simulink model "emrax_speed_control_mode"  (R2022b)
settings: Solver=FixedStepAuto  StartTime=0.0  StopTime=2  FixedStep=1e-4  RelTol=1e-3
values from neighbouring files (symbols this model uses):
  a_fw = log(9)/trfw    [emrax_sim.m]
  ba = 2*k^2*(as*J - bm)/(np^2*psi)    [emrax_sim.m]
  bm = 0.008    [emrax_sim.m]
  I_max = I_base    [emrax_sim.m]
  J = 421e-4    (= 0.0421)    [emrax_sim.m]
  k = 1    [emrax_sim.m]
  ki_d = (ac^2)*Ld    [emrax_sim.m]
  ki_q = (ac^2)*Lq    [emrax_sim.m]
  ki_s = 2*k^2*as^2*J/(np^2*psi)    [emrax_sim.m]
  kp_d = ac*Ld    [emrax_sim.m]
  kp_q = ac*Lq    [emrax_sim.m]
  kp_s = 2*k^2*as*J/(np^2*psi)    [emrax_sim.m]
  Ld = 177*10^(-6)    (= 0.000177)    [emrax_sim.m]
  Lq = 183*10^(-6)    (= 0.000183)    [emrax_sim.m]
  max_temp = 140    [emrax_sim.m]
  np = 10    [emrax_sim.m]
  Peak_power = 50000    [emrax_sim.m]
  Peak_regen = -1500000    [emrax_sim.m]
  psi = 0.0542*k    (= 0.0542)    [emrax_sim.m]
  Ra_d = ac*Ld-Rs    [emrax_sim.m]
  Ra_q = ac*Lq-Rs    [emrax_sim.m]
  rpm_nom = 5100    [emrax_sim.m]
  Rs = 18e-3    (= 0.018)    [emrax_sim.m]
  temp_threshold = 100    [emrax_sim.m]
  u_dc = 550    [emrax_sim.m]
  u_nom = u_dc*k    (= 550)    [emrax_sim.m]
  Vd_lim = u_nom    (= 550)    [emrax_sim.m]
libraries: simulink x6, spsMeanLib x1, spspowerguiLib x1
settings Model: Creator=alexa  LastModifiedBy=alexa

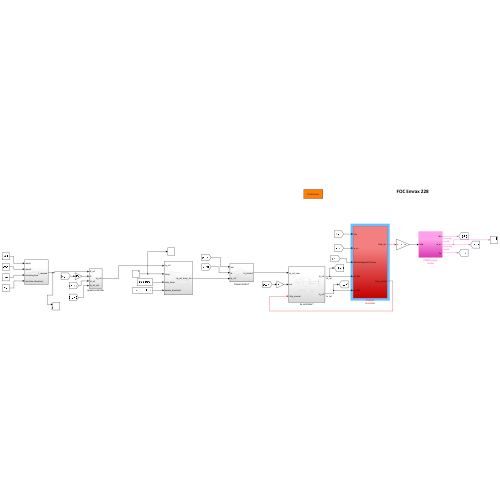
[thumbnail: Simulink's stored preview of the top-level diagram]
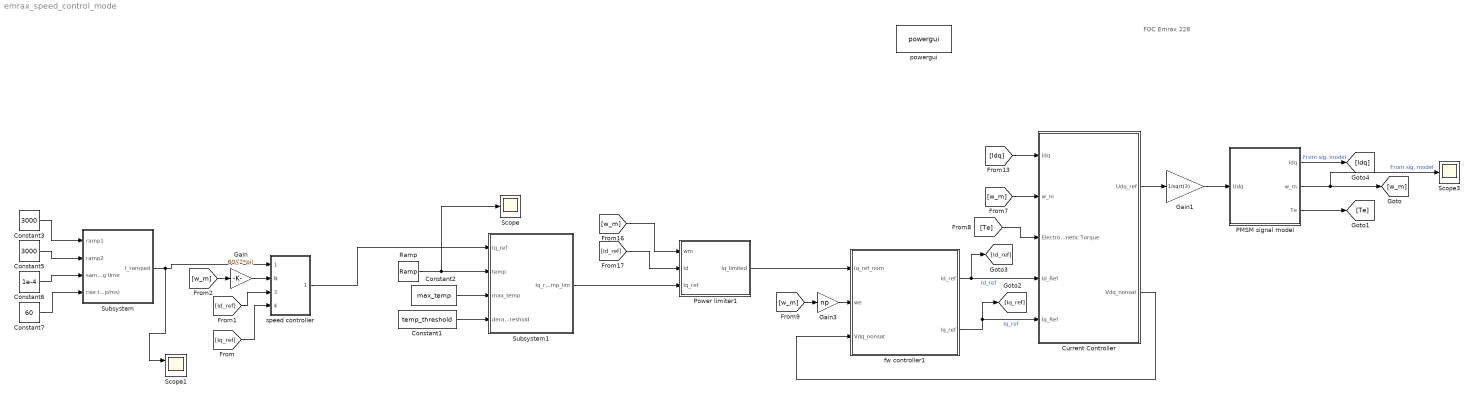
== system emrax_speed_control_mode ==
  note: FOC Emrax 228
  Constant1 : Constant  Value=temp_threshold
  Constant2 : Constant  Value=max_temp
  Constant3 : Constant  Value=3000
  Constant5 : Constant  Value=3000
  Constant6 : Constant  Value=1e-4
  Constant7 : Constant  Value=60
  Current Controller : Subsystem
  Gain : Gain  Gain=60/(2*pi)
  Gain1 : Gain  Gain=1/sqrt(3)
  Gain3 : Gain  Gain=np
  PMSM signal model : Subsystem
  Power limiter1 : Subsystem
  Ramp : simulink/Sources/Ramp  slope=1  start=0  InitialOutput=30
  Scope : Scope
  Scope1 : Scope  NumInputPorts=2
  Scope3 : Scope
  Subsystem : Subsystem
  Subsystem1 : Subsystem
  fw controller1 : Subsystem
  powergui : spspowerguiLib/powergui  Priority=1  SimulationMode=Continuous  SampleTime=50e-6  frequency=60  Iterations=50  frequencyindice=0  Pbase=100e6  ErrMax=1e-4  UnitsV=kV  UnitsW=MW  buscounter=0  FunctionMessages=off  echomessages=off  EnableUseOfTLC=off  CurrentSourceSwitches=off  DisableSnubberDevices=off  DisableRonSwitches=off  DisableVfSwitches=off  DisplayEquations=off  AutomaticDiscreteSolvers=off  SolverType=Tustin/Backward Euler (TBE)  Interpol=off  ExternalGateDelay=off  methode=off  Ts=100  x0status=blocks  SPID=on  SwTol=0  HookPort=off  NonlinearTolerance=0  nMaxIteration=15  ContinueOnMaxIteration=off  RestoreLinks=warning  ResistiveCurrentMeasurement=off  Frange=[0:2:500]  Ylog=off  Xlog=on  ShowGrid=off  save=off  variable=ZData  structure=0  ZoomFFT=off  StartTime=0.0  cycles=1  DisplayStyle=1  fundamental=60  FreqAxis=off  MaxFrequency=1000  frequencyindicesteady=1  RmsSteady=1  display=off
  speed controller : Subsystem
  wires:
  fw controller1/2(Iq_ref) -> Current Controller/5(Iq_Ref), [Iq_ref]  "Iq_ref"
  Gain3/1 -> fw controller1/2(we)
  Constant7/1 -> Subsystem/4(rise time (Amp/ms))
  Constant6/1 -> Subsystem/3(sampling time)
  PMSM signal model/3("Te ") -> [Te]
  [Te] -> Current Controller/3(Electromagnetic Torque)
  [w_m] -> Gain3/1
  [w_m] -> Current Controller/2(w_m)
  PMSM signal model/1(Idq) -> [Idq]  "From sig. model"
  Gain1/1 -> PMSM signal model/1(Udq)
  Constant5/1 -> Subsystem/2(ramp2)
  Current Controller/2(Vdq_nonsat) -> fw controller1/3(Vdq_nonsat)
  [Idq] -> Current Controller/1(Idq)
  fw controller1/1(Id_ref) -> Current Controller/4(Id_Ref), [Id_ref]  "Id_ref"
  Current Controller/1("Udq_ref ") -> Gain1/1
  PMSM signal model/2("w_m ") -> [w_m], Scope3/1  "From sig. model"
  Constant3/1 -> Subsystem/1(ramp1)
  [w_m] -> Power limiter1/1(wm)
  [Id_ref] -> Power limiter1/2(Id)
  [Iq_ref] -> speed controller/4(Iq_ref_sat)
  [Id_ref] -> speed controller/3(Id_ref)
  Gain/1 -> speed controller/2(N)
  [w_m] -> Gain/1
  Power limiter1/1(Iq_limited) -> fw controller1/1(Iq_ref_nom)
  Constant1/1 -> Subsystem1/4(derate_threshold)
  Constant2/1 -> Subsystem1/3(max_temp)
  Ramp/1 -> Scope/1, Subsystem1/2(temp)
  Subsystem1/1(Iq_ref_temp_lim) -> Power limiter1/3(Iq_ref)
  speed controller/1(Iq_ref) -> Subsystem1/1(Iq_ref)
  Subsystem/1(I_ramped) -> Scope1/1, speed controller/1(N_ref)

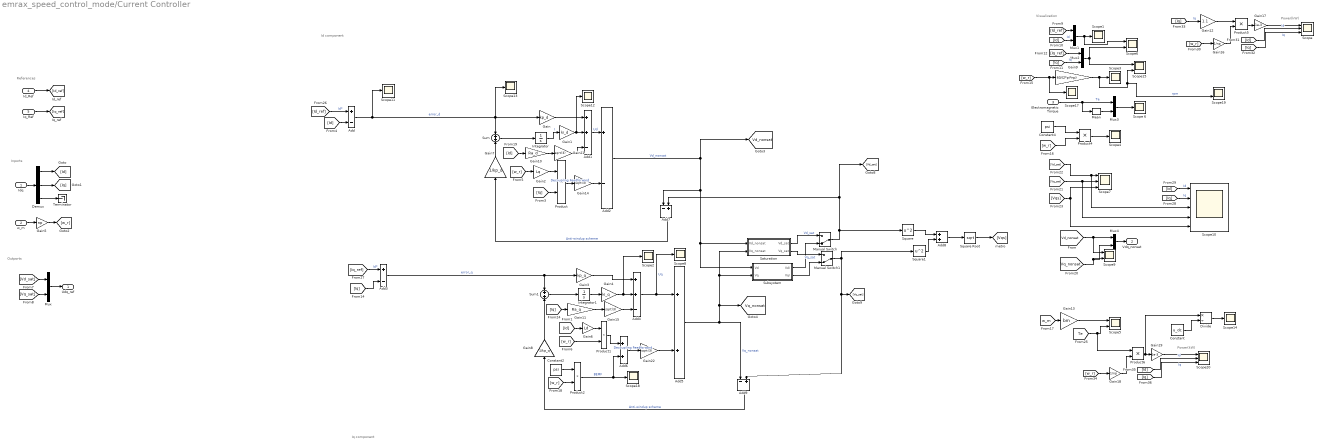
== system emrax_speed_control_mode/Current Controller ==
  note: Power(kW)
  note: References
  note: Id component
  note: Iq component
  note: Inports
  note: Outports
  note: Visualization
  note: Power(kW)
  Idq : Inport
  w_m : Inport  Port=2
  Electromagnetic Torque : Inport  Port=3
  Id_Ref : Inport  Port=4
  Iq_Ref : Inport  Port=5
  Add : Sum  Inputs=+-
  Add1 : Sum  Inputs=++-
  Add2 : Sum  Inputs=+-
  Add3 : Sum  Inputs=+-
  Add4 : Sum  Inputs=++-
  Add5 : Sum
  Add6 : Sum
  Add7 : Sum  Inputs=-+
  Add8 : Sum
  Add9 : Sum  Inputs=-+
  Constant : Constant  Value=u_dc
  Constant2 : Constant  Value=psi
  Constant4 : Constant  Value=psi
  Demux : Demux  Outputs=3
  Divide : Product  Inputs=*/
  Gain : Gain  Gain=kp_d
  Gain1 : Gain  Gain=ki_d
  Gain10 : Gain  Gain=Ra_d
  Gain11 : Gain  Gain=Ra_q
  Gain12 : Gain  Gain=1.1
  Gain13 : Gain  Gain=bm
  Gain{14..15,21..22} (4 alike) : Gain  Gain=sqrt(3)
  Gain16 : Gain  Gain=1/np
  Gain17 : Gain  Gain=1e-3
  Gain18 : Gain  Gain=1/np
  Gain19 : Gain  Gain=1e-3
  Gain2 : Gain  Gain=Lq
  Gain3 : Gain  Gain=kp_q
  Gain4 : Gain  Gain=ki_q
  Gain5 : Gain  Gain=np
  Gain6 : Gain  Gain=Ld
  Gain7 : Gain  Gain=1/kp_d
  Gain8 : Gain  Gain=1/kp_q
  Gain9 : Gain  Gain=60/(2*pi*np)
  Integrator : Integrator
  Integrator1 : Integrator
  Manual Switch : ManualSwitch  CurrentSetting=0
  Manual Switch1 : ManualSwitch  CurrentSetting=0
  Mean : spsMeanLib/Mean  Freq=fsw  Vinit=0  Ts=0
  Mux{,1..4} (5 alike) : Mux  Inputs=2
  Product{,1..2,4..6} (6 alike) : Product
  Saturation : Subsystem
  Scope : Scope  NumInputPorts=3
  Scope 6 : Scope
  Scope{1..4,8,11..14,17..18} (11 alike) : Scope
  Scope10 : Scope  NumInputPorts=5
  Scope{5..6,9,15,19} (5 alike) : Scope  NumInputPorts=2
  Scope20 : Scope  NumInputPorts=3
  Scope7 : Scope  NumInputPorts=3
  Square : Math  Operator=square
  Square Root : Sqrt
  Square1 : Math  Operator=square
  Subsystem : Subsystem
  Sum : Sum
  Sum1 : Sum
  Terminator : Terminator
  "Udq_ref " : Outport  VectorParamsAs1DForOutWhenUnconnected=off
  Vdq_nonsat : Outport  Port=2
  tag scope: Vd_nonsat=global, Vq_nonsat=global
  wires:
  Gain4/1 -> Scope2/1, Add4/2
  [Id] -> Gain6/1
  Add4/1 -> Scope8/1, Add5/1  "Uq"
  Add1/1 -> Add2/1  "Ud"
  [w_r] -> Gain2/1
  Gain2/1 -> Product/1
  Gain3/1 -> Add4/1
  [Iq] -> Product/2
  Integrator/1 -> Gain1/1  "I"
  Sum/1 -> Integrator/1
  Gain/1 -> Add1/1
  [w_r] -> Product1/2
  Gain6/1 -> Product1/1
  Idq/1 -> Demux/1
  Product/1 -> Gain14/1  "Decoupling Feedforward"
  Gain7/1 -> Sum/2
  Add2/1 -> [Vd_nonsat], Saturation/1(Vd_nonsat), Subsystem/1(Vd), Add7/1  "Vd_nonsat"
  Add7/1 -> Gain7/1  "Anti-windup scheme"
  Sum1/1 -> Integrator1/1
  Add5/1 -> Add9/1, Subsystem/2(Vq), Saturation/2(Vq_nonsat), [Vq_nonsat]  "Vq_nonsat"
  Gain8/1 -> Sum1/2
  Add9/1 -> Gain8/1  "Anti-windup scheme"
  Demux/1 -> [Id]
  Demux/2 -> [Iq]
  Demux/3 -> Terminator/1
  w_m/1 -> Gain5/1
  Gain5/1 -> [w_r]
  [Vd_sat] -> Mux/1
  [Vq_sat] -> Mux/2
  Mux/1 -> "Udq_ref "/1
  [Id] -> Add/2
  Mux1/1 -> Scope6/1, Scope1/1
  [Id_ref] -> Mux1/1
  [Id] -> Mux1/2  "Id"
  [Iq_ref] -> Mux2/1
  [Iq] -> Mux2/2  "Iq"
  [w_r] -> Scope17/1, Gain9/1
  Gain9/1 -> Scope19/2, Scope15/2, Scope3/1  "rpm"
  Mux3/1 -> Scope 6/1
  Electromagnetic Torque/1 -> Mean/1, Mux3/1  "Te"
  Mean/1 -> Mux3/2
  Constant2/1 -> Product2/1
  Product1/1 -> Add6/1
  Add6/1 -> Gain22/1  "Decoupling Feedforward"
  Add/1 -> Scope11/1, Gain/1, Sum/1, Scope13/1  "error_d"
  Add3/1 -> Sum1/1, Gain3/1  "error_q"
  [Iq] -> Add3/2
  Gain1/1 -> Scope12/1, Add1/2
  Integrator1/1 -> Gain4/1
  Square1/1 -> Add8/2
  Square/1 -> Add8/1
  Add8/1 -> Square Root/1
  [Vd_nonsat] -> Scope9/1, Mux4/1
  [Vq_nonsat] -> Mux4/2, Scope9/2
  Square Root/1 -> [Vqs]
  [Vd_sat] -> Scope10/3, Scope7/1
  [Vq_sat] -> Scope10/4, Scope7/2
  [Vqs] -> Scope7/3, Scope10/5
  [Id] -> Gain10/1
  [Iq] -> Gain11/1
  [w_r] -> Product4/2
  Constant4/1 -> Product4/1
  Product4/1 -> Scope4/1
  Id_Ref/1 -> [Id_ref]
  Iq_Ref/1 -> [Iq_ref]
  Gain13/1 -> Scope5/1
  [Te] -> Product6/1, Scope5/2
  [w_m] -> Gain13/1
  Gain12/1 -> Product5/1
  Mux2/1 -> Scope6/2, Scope15/1
  [Iq] -> Scope10/2  "Iq"
  [Id] -> Scope10/1  "Id"
  [Id_ref] -> Add/1  "Id*"
  Subsystem/1(Vd\) -> Manual Switch/2
  Saturation/1(Vd_sat) -> Manual Switch/1  "Vd_sat"
  Saturation/2(Vq_sat) -> Manual Switch1/1  "Vq_sat"
  Subsystem/2(Vq\) -> Manual Switch1/2
  Manual Switch/1 -> Square/1, [Vd_sat], Add7/2
  Manual Switch1/1 -> [Vq_sat], Add9/2, Square1/1
  Gain11/1 -> Gain15/1
  [w_r] -> Product2/2
  Product2/1 -> Scope18/1, Add6/2  "BEMF"
  Mux4/1 -> Vdq_nonsat/1
  [Iq_ref] -> Add3/1  "Id*"
  Product5/1 -> Gain17/1
  [w_r] -> Gain16/1
  Gain16/1 -> Product5/2
  [Id] -> Scope/2  "Id"
  [Iq] -> Scope/3  "Iq"
  [Iq] -> Gain12/1  "Iq"
  Gain17/1 -> Scope/1
  Gain19/1 -> Scope20/1
  [Iq] -> Scope20/3  "Iq"
  [Id] -> Scope20/2  "Id"
  Gain18/1 -> Product6/2
  Product6/1 -> Divide/1, Gain19/1
  [w_r] -> Gain18/1
  Gain15/1 -> Add4/3
  Gain10/1 -> Gain21/1
  Gain21/1 -> Add1/3
  Gain14/1 -> Add2/2
  Gain22/1 -> Add5/2
  Constant/1 -> Divide/2
  Divide/1 -> Scope14/1

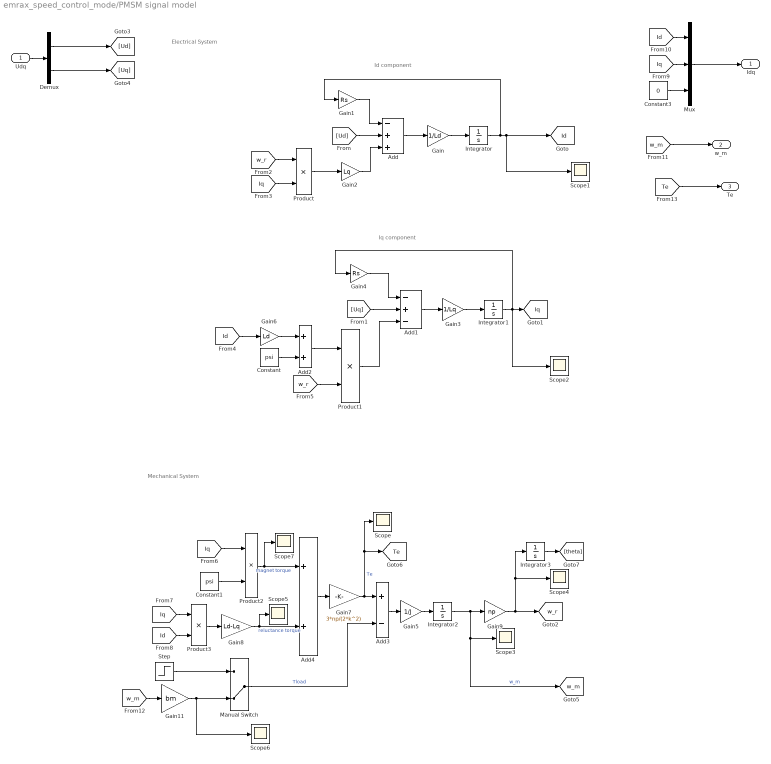
== system emrax_speed_control_mode/PMSM signal model ==
  note: Electrical System
  note: Id component
  note: Iq component
  note: Mechanical System
  Udq : Inport
  Add : Sum  Inputs=-++
  Add1 : Sum  Inputs=-+-
  Add2 : Sum
  Add3 : Sum  Inputs=+-
  Add4 : Sum
  Constant : Constant  Value=psi
  Constant1 : Constant  Value=psi
  Constant3 : Constant  Value=0
  Demux : Demux  Outputs=2
  Gain : Gain  Gain=1/Ld
  Gain1 : Gain  Gain=Rs
  Gain11 : Gain  Gain=bm
  Gain2 : Gain  Gain=Lq
  Gain3 : Gain  Gain=1/Lq
  Gain4 : Gain  Gain=Rs
  Gain5 : Gain  Gain=1/J
  Gain6 : Gain  Gain=Ld
  Gain7 : Gain  Gain=3*np/(2*k^2)
  Gain8 : Gain  Gain=Ld-Lq
  Gain9 : Gain  Gain=np
  Integrator{,1..3} (4 alike) : Integrator
  Manual Switch : ManualSwitch  CurrentSetting=0
  Mux : Mux  Inputs=3
  Product{,1..3} (4 alike) : Product
  Scope{,1..7} (8 alike) : Scope
  Step : Step  Time=0.5  After=200  SampleTime=0
  Idq : Outport  VectorParamsAs1DForOutWhenUnconnected=off
  "w_m " : Outport  Port=2  VectorParamsAs1DForOutWhenUnconnected=off
  "Te " : Outport  Port=3  VectorParamsAs1DForOutWhenUnconnected=off
  tag scope: Id=global, Iq=global, Te=global, w_m=global, w_r=global
  wires:
  Add3/1 -> Gain5/1
  Add2/1 -> Product1/1
  Product/1 -> Gain2/1
  Gain/1 -> Integrator/1
  Integrator1/1 -> Scope2/1, [Iq], Gain4/1
  Gain6/1 -> Add2/1
  Gain1/1 -> Add/1
  Product3/1 -> Gain8/1
  Integrator/1 -> Gain1/1, Scope1/1, [Id]
  Gain8/1 -> Add4/2, Scope5/1  "reluctance torque"
  Gain5/1 -> Integrator2/1
  Gain7/1 -> Add3/1, [Te], Scope/1  "Te"
  Constant1/1 -> Product2/2
  Add4/1 -> Gain7/1
  [Iq] -> Product3/1
  Product2/1 -> Add4/1, Scope7/1  "magnet torque"
  [Iq] -> Product2/1
  Gain2/1 -> Add/3
  [w_r] -> Product/1
  [Id] -> Gain6/1
  [Iq] -> Product/2
  Gain3/1 -> Integrator1/1
  [w_r] -> Product1/2
  Constant/1 -> Add2/2
  Gain4/1 -> Add1/1
  Product1/1 -> Add1/3
  Add1/1 -> Gain3/1
  [Ud] -> Add/2
  Add/1 -> Gain/1
  [Uq] -> Add1/2
  [Id] -> Product3/2
  Udq/1 -> Demux/1
  Integrator2/1 -> Gain9/1, [w_m], Scope3/1  "w_m"
  Gain9/1 -> Scope4/1, Integrator3/1, [w_r]
  Manual Switch/1 -> Add3/2  "Tload"
  Step/1 -> Manual Switch/1
  [w_m] -> Gain11/1
  [Id] -> Mux/1
  [Iq] -> Mux/2
  [w_m] -> "w_m "/1
  Constant3/1 -> Mux/3
  [Te] -> "Te "/1
  Integrator3/1 -> [theta]
  Demux/1 -> [Ud]
  Demux/2 -> [Uq]
  Mux/1 -> Idq/1
  Gain11/1 -> Scope6/1, Manual Switch/2

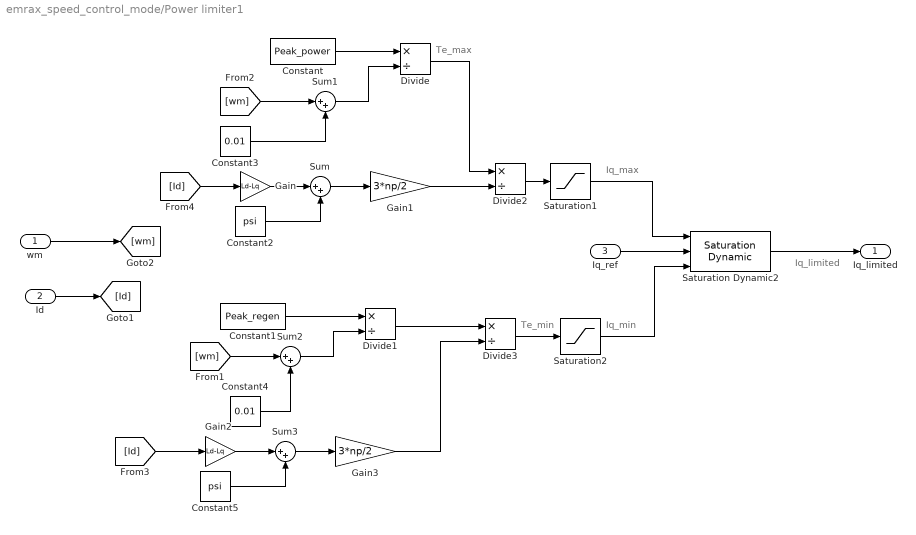
== system emrax_speed_control_mode/Power limiter1 ==
  note: Te_max
  note: Iq_limited
  note: Iq_max
  note: Iq_min
  note: Te_min
  wm : Inport
  Id : Inport  Port=2
  Iq_ref : Inport  Port=3
  Constant : Constant  Value=Peak_power
  Constant1 : Constant  Value=Peak_regen
  Constant2 : Constant  Value=psi
  Constant3 : Constant  Value=0.01
  Constant4 : Constant  Value=0.01
  Constant5 : Constant  Value=psi
  Divide{,1..3} (4 alike) : Product  Inputs=*/
  Gain : Gain  Gain=Ld-Lq
  Gain1 : Gain  Gain=3*np/2
  Gain2 : Gain  Gain=Ld-Lq
  Gain3 : Gain  Gain=3*np/2
  Saturation Dynamic2 : simulink/Discontinuities/Saturation Dynamic  OutMin=[]  OutMax=[]  OutDataTypeStr=Inherit: Same as second input  OutDataType=fixdt(1, 16)  OutScaling=2^-10  DoSatur=off
  Saturation1 : Saturate  UpperLimit=10000  LowerLimit=-10000
  Saturation2 : Saturate  UpperLimit=10000  LowerLimit=-10000
  Sum{,1..3} (4 alike) : Sum  Inputs=|++
  Iq_limited : Outport
  wires:
  Sum2/1 -> Divide1/2
  [wm] -> Sum2/1
  Constant4/1 -> Sum2/2
  Saturation2/1 -> Saturation Dynamic2/3
  Saturation1/1 -> Saturation Dynamic2/1
  Constant3/1 -> Sum1/2
  [wm] -> Sum1/1
  Sum1/1 -> Divide/2
  Divide2/1 -> Saturation1/1
  Divide3/1 -> Saturation2/1
  Divide/1 -> Divide2/1
  Constant1/1 -> Divide1/1
  Constant/1 -> Divide/1
  Divide1/1 -> Divide3/1
  Saturation Dynamic2/1 -> Iq_limited/1
  wm/1 -> [wm]
  Iq_ref/1 -> Saturation Dynamic2/2
  Gain1/1 -> Divide2/2
  Gain/1 -> Sum/1
  Constant2/1 -> Sum/2
  Sum/1 -> Gain1/1
  Sum3/1 -> Gain3/1
  [Id] -> Gain2/1
  Gain2/1 -> Sum3/1
  Constant5/1 -> Sum3/2
  Gain3/1 -> Divide3/2
  Id/1 -> [Id]
  [Id] -> Gain/1

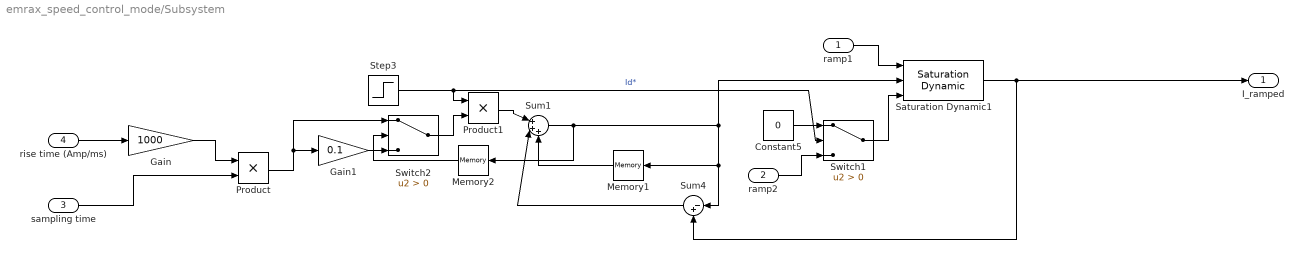
== system emrax_speed_control_mode/Subsystem ==
  ramp1 : Inport
  ramp2 : Inport  Port=2
  sampling time : Inport  Port=3
  rise time (Amp/ms) : Inport  Port=4
  Constant5 : Constant  Value=0
  Gain : Gain  Gain=1000
  Gain1 : Gain  Gain=0.1
  Memory1 : Memory
  Memory2 : Memory
  Product : Product
  Product1 : Product
  Saturation Dynamic1 : simulink/Discontinuities/Saturation Dynamic  OutMin=[]  OutMax=[]  OutDataTypeStr=Inherit: Same as second input  OutDataType=fixdt(1, 16)  OutScaling=2^-10  DoSatur=off
  Step3 : Step  Time=2  Before=1  After=-1  SampleTime=0
  Sum1 : Sum  Inputs=|+++
  Sum4 : Sum  Inputs=|-+
  Switch1 : Switch  Criteria=u2 > Threshold  SaturateOnIntegerOverflow=off  InputSameDT=off
  Switch2 : Switch  Criteria=u2 > Threshold  SaturateOnIntegerOverflow=off  InputSameDT=off
  I_ramped : Outport
  wires:
  Sum1/1 -> Memory2/1, Sum4/1, Memory1/1, Saturation Dynamic1/2
  Switch2/1 -> Product1/2
  Memory2/1 -> Switch2/2
  Product1/1 -> Sum1/1
  Memory1/1 -> Sum1/3
  Gain1/1 -> Switch2/3
  Switch1/1 -> Saturation Dynamic1/3
  Step3/1 -> Switch1/2, Product1/1  "Id*"
  Sum4/1 -> Sum1/2
  Constant5/1 -> Switch1/1
  Saturation Dynamic1/1 -> Sum4/2, I_ramped/1
  ramp2/1 -> Switch1/3
  ramp1/1 -> Saturation Dynamic1/1
  rise time (Amp/ms)/1 -> Gain/1
  sampling time/1 -> Product/2
  Gain/1 -> Product/1
  Product/1 -> Switch2/1, Gain1/1

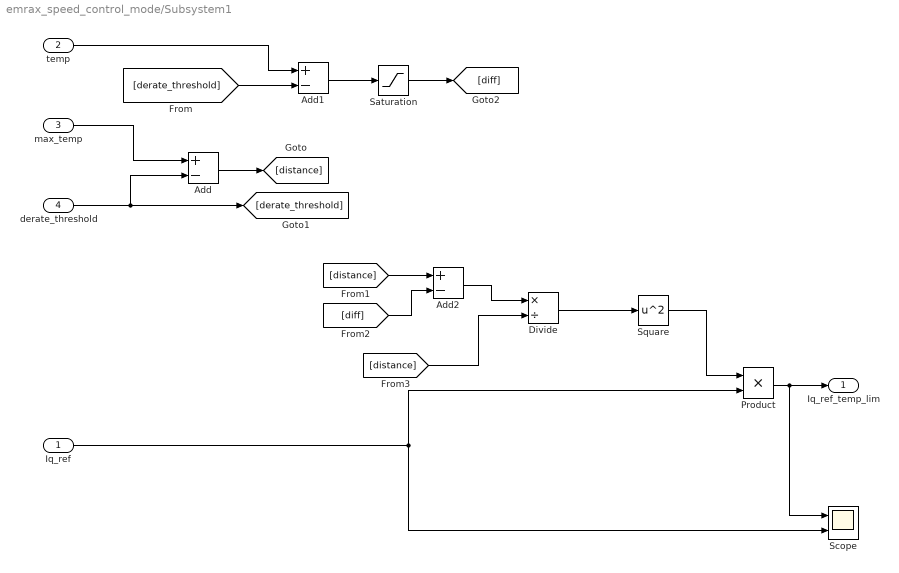
== system emrax_speed_control_mode/Subsystem1 ==
  Iq_ref : Inport
  temp : Inport  Port=2
  max_temp : Inport  Port=3
  derate_threshold : Inport  Port=4
  Add : Sum  Inputs=+-
  Add1 : Sum  Inputs=+-
  Add2 : Sum  Inputs=+-
  Divide : Product  Inputs=*/
  Product : Product
  Saturation : Saturate  UpperLimit=1000  LowerLimit=0
  Scope : Scope  NumInputPorts=2
  Square : Math  Operator=square
  Iq_ref_temp_lim : Outport
  wires:
  max_temp/1 -> Add/1
  Add/1 -> [distance]
  derate_threshold/1 -> [derate_threshold], Add/2
  [derate_threshold] -> Add1/2
  temp/1 -> Add1/1
  Add1/1 -> Saturation/1
  Saturation/1 -> [diff]
  [distance] -> Add2/1
  [diff] -> Add2/2
  Add2/1 -> Divide/1
  [distance] -> Divide/2
  Divide/1 -> Square/1
  Iq_ref/1 -> Product/2, Scope/2
  Square/1 -> Product/1
  Product/1 -> Scope/1, Iq_ref_temp_lim/1

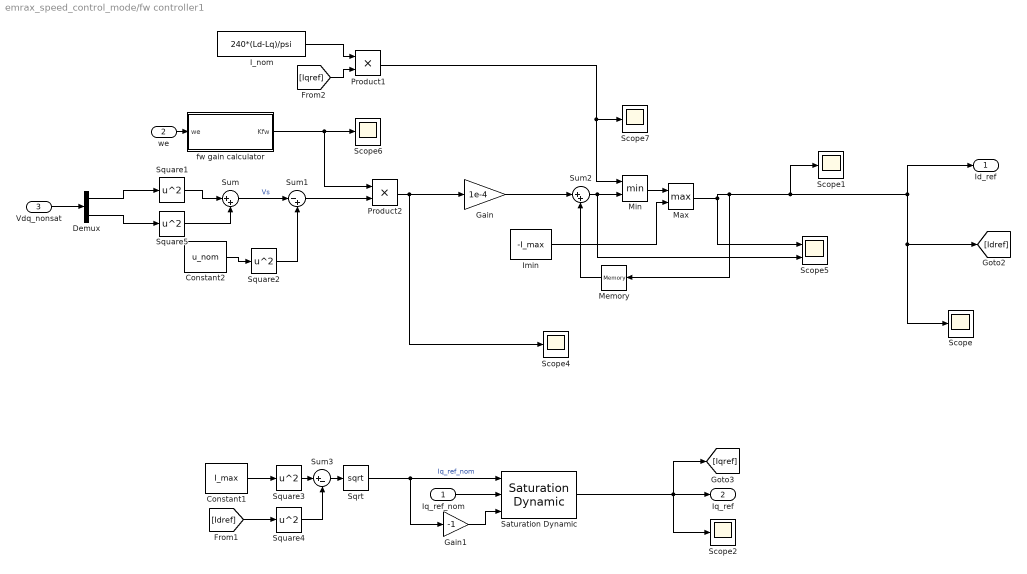
== system emrax_speed_control_mode/fw controller1 ==
  Iq_ref_nom : Inport
  we : Inport  Port=2
  Vdq_nonsat : Inport  Port=3
  Constant1 : Constant  Value=I_max
  Constant2 : Constant  Value=u_nom
  Demux : Demux  Outputs=2
  Gain : Gain  Gain=1e-4
  Gain1 : Gain  Gain=-1
  I_nom : Constant  Value=240*(Ld-Lq)/psi
  Imin : Constant  Value=-I_max
  Max : MinMax  Function=max  Inputs=2
  Memory : Memory
  Min : MinMax  Inputs=2
  Product1 : Product
  Product2 : Product
  Saturation Dynamic : simulink/Discontinuities/Saturation Dynamic  OutMin=[]  OutMax=[]  OutDataTypeStr=Inherit: Same as second input  OutDataType=fixdt(1, 16)  OutScaling=2^-10  DoSatur=off
  Scope{,1..2,4,6..7} (6 alike) : Scope
  Scope5 : Scope  NumInputPorts=2
  Sqrt : Sqrt
  Square{1..5} (5 alike) : Math  Operator=square
  Sum : Sum  Inputs=|++
  Sum1 : Sum  Inputs=|-+
  Sum2 : Sum  Inputs=|++
  Sum3 : Sum  Inputs=|+-
  fw gain calculator : Subsystem
  Id_ref : Outport
  Iq_ref : Outport  Port=2
  wires:
  Max/1 -> Scope5/1, Memory/1, Scope1/1, [Idref], Scope/1, Id_ref/1
  Product2/1 -> Scope4/1, Gain/1
  Sum1/1 -> Product2/2
  fw gain calculator/1(Kfw) -> Scope6/1, Product2/1
  [Iqref] -> Product1/2
  [Idref] -> Square4/1
  Square5/1 -> Sum/2
  Square1/1 -> Sum/1
  Vdq_nonsat/1 -> Demux/1
  Demux/1 -> Square1/1
  Demux/2 -> Square5/1
  I_nom/1 -> Product1/1
  Gain1/1 -> Saturation Dynamic/3
  Imin/1 -> Max/2
  Sum3/1 -> Sqrt/1
  Constant2/1 -> Square2/1
  Sum/1 -> Sum1/1  "Vs"
  Square2/1 -> Sum1/2
  we/1 -> fw gain calculator/1(we)
  Constant1/1 -> Square3/1
  Square3/1 -> Sum3/1
  Square4/1 -> Sum3/2
  Iq_ref_nom/1 -> Saturation Dynamic/2
  Sqrt/1 -> Saturation Dynamic/1, Gain1/1  "Iq_ref_nom"
  Saturation Dynamic/1 -> Scope2/1, Iq_ref/1, [Iqref]
  Gain/1 -> Sum2/1
  Sum2/1 -> Min/2, Scope5/2
  Memory/1 -> Sum2/2
  Product1/1 -> Min/1, Scope7/1
  Min/1 -> Max/1

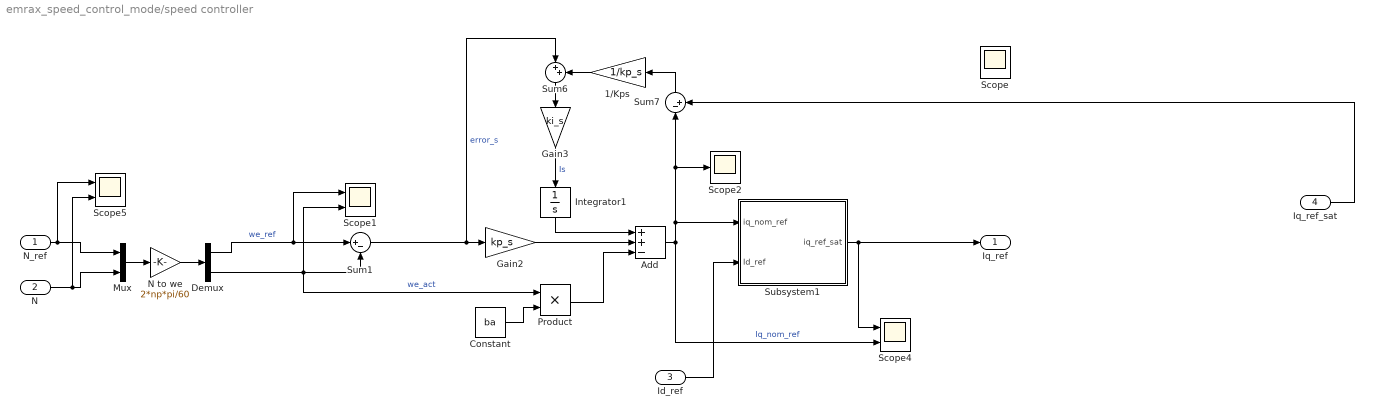
== system emrax_speed_control_mode/speed controller ==
  N_ref : Inport
  N : Inport  Port=2
  Id_ref : Inport  Port=3
  Iq_ref_sat : Inport  Port=4
  1/Kps : Gain  Gain=1/kp_s
  Add : Sum  Inputs=++-
  Constant : Constant  Value=ba
  Demux : Demux  Outputs=2
  Gain2 : Gain  Gain=kp_s
  Gain3 : Gain  Gain=ki_s
  Integrator1 : Integrator
  Mux : Mux  Inputs=2
  N to we : Gain  Gain=2*np*pi/60
  Product : Product
  Scope : Scope
  Scope1 : Scope  NumInputPorts=2
  Scope2 : Scope
  Scope4 : Scope  NumInputPorts=2
  Scope5 : Scope  NumInputPorts=2
  Subsystem1 : Subsystem
  Sum1 : Sum  Inputs=|+-
  Sum6 : Sum  Inputs=|++
  Sum7 : Sum  Inputs=|-+
  Iq_ref : Outport
  wires:
  Sum7/1 -> 1/Kps/1
  Add/1 -> Scope2/1, Sum7/1, Subsystem1/1(iq_nom_ref), Scope4/2  "Iq_nom_ref"
  Gain2/1 -> Add/2
  1/Kps/1 -> Sum6/2
  Sum1/1 -> Gain2/1, Sum6/1  "error_s"
  N_ref/1 -> Scope5/1, Mux/1
  N/1 -> Scope5/2, Mux/2
  Constant/1 -> Product/2
  Gain3/1 -> Integrator1/1  "Is"
  Product/1 -> Add/3
  Demux/1 -> Scope1/1, Sum1/1  "we_ref"
  Demux/2 -> Product/1, Sum1/2, Scope1/2  "we_act"
  Sum6/1 -> Gain3/1
  Subsystem1/1(iq_ref_sat) -> Scope4/1, Iq_ref/1
  Mux/1 -> N to we/1
  N to we/1 -> Demux/1
  Integrator1/1 -> Add/1
  Id_ref/1 -> Subsystem1/2(Id_ref)
  Iq_ref_sat/1 -> Sum7/2

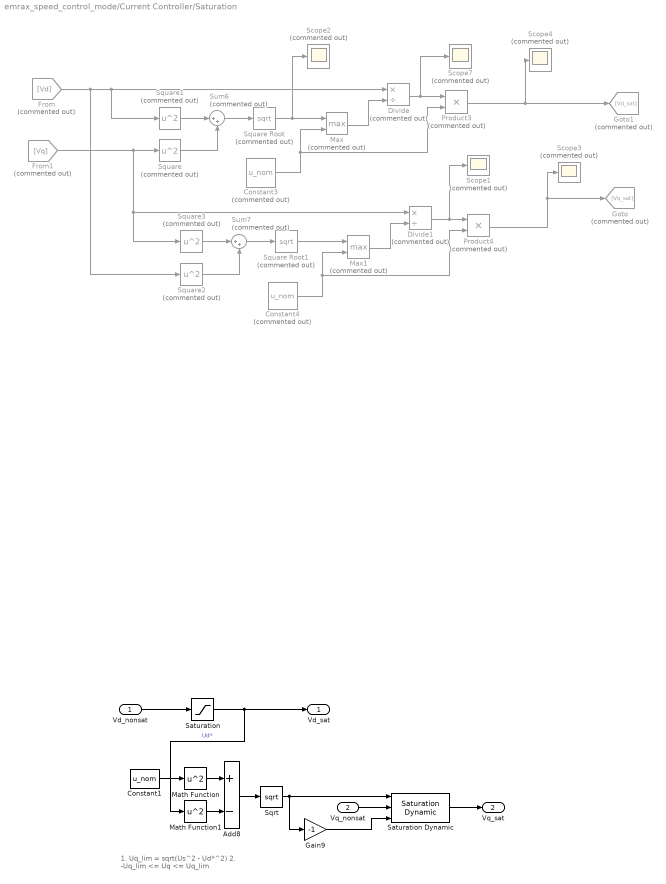
== system emrax_speed_control_mode/Current Controller/Saturation ==
  note: 1. Uq_lim = sqrt(Us^2 - Ud*^2)
      |
      | 2. -Uq_lim <= Uq <= Uq_lim
  Vd_nonsat : Inport
  Vq_nonsat : Inport  Port=2
  Add8 : Sum  Inputs=+-
  Constant1 : Constant  Value=u_nom
  Constant3 : Constant  Commented=on  Value=u_nom
  Constant4 : Constant  Commented=on  Value=u_nom
  Divide : Product  Commented=on  Inputs=*/
  Divide1 : Product  Commented=on  Inputs=*/
  From : From  Commented=on  GotoTag=Vd
  From1 : From  Commented=on  GotoTag=Vq
  Gain9 : Gain  Gain=-1
  Goto : Goto  Commented=on  GotoTag=Vq_sat
  Goto1 : Goto  Commented=on  GotoTag=Vd_sat
  Math Function : Math  Operator=square  SignedPower=on
  Math Function1 : Math  Operator=square  SignedPower=on
  Max : MinMax  Commented=on  Function=max  Inputs=2
  Max1 : MinMax  Commented=on  Function=max  Inputs=2
  Product3 : Product  Commented=on
  Product4 : Product  Commented=on
  Saturation : Saturate  UpperLimit=Vd_lim  LowerLimit=-Vd_lim  LinearizeAsGain=off
  Saturation Dynamic : simulink/Discontinuities/Saturation Dynamic  OutMin=[]  OutMax=[]  OutDataTypeStr=Inherit: Same as second input  OutDataType=fixdt(1, 16)  OutScaling=2^-10  DoSatur=off
  Scope{1..4,7} (5 alike) : Scope  Commented=on
  Sqrt : Sqrt
  Square{,1..3} (4 alike) : Math  Commented=on  Operator=square
  Square Root : Sqrt  Commented=on
  Square Root1 : Sqrt  Commented=on
  Sum6 : Sum  Commented=on  Inputs=|++
  Sum7 : Sum  Commented=on  Inputs=|++
  Vd_sat : Outport
  Vq_sat : Outport  Port=2
  wires:
  From/1 -> Square2/1, Divide/1, Square1/1
  Divide/1 -> Scope7/1, Product3/1
  Constant4/1 -> Product4/2, Max1/2
  Square1/1 -> Sum6/1
  Square3/1 -> Sum7/1
  Divide1/1 -> Scope1/1, Product4/1
  Constant3/1 -> Product3/2, Max/2
  Square2/1 -> Sum7/2
  Sum6/1 -> Square Root/1
  Square/1 -> Sum6/2
  From1/1 -> Divide1/1, Square3/1, Square/1
  Sum7/1 -> Square Root1/1
  Product3/1 -> Goto1/1, Scope4/1
  Max/1 -> Divide/2
  Square Root/1 -> Scope2/1, Max/1
  Square Root1/1 -> Max1/1
  Max1/1 -> Divide1/2
  Vd_nonsat/1 -> Saturation/1
  Saturation/1 -> Math Function1/1, Vd_sat/1  "Ud*"
  Math Function/1 -> Add8/1
  Math Function1/1 -> Add8/2
  Gain9/1 -> Saturation Dynamic/3
  Add8/1 -> Sqrt/1
  Sqrt/1 -> Gain9/1, Saturation Dynamic/1
  Constant1/1 -> Math Function/1
  Vq_nonsat/1 -> Saturation Dynamic/2
  Saturation Dynamic/1 -> Vq_sat/1
  Product4/1 -> Goto/1, Scope3/1

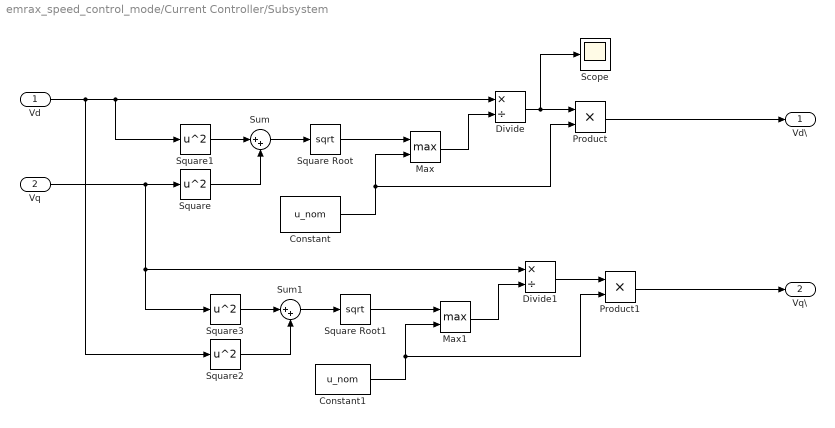
== system emrax_speed_control_mode/Current Controller/Subsystem ==
  Vd : Inport
  Vq : Inport  Port=2
  Constant : Constant  Value=u_nom
  Constant1 : Constant  Value=u_nom
  Divide : Product  Inputs=*/
  Divide1 : Product  Inputs=*/
  Max : MinMax  Function=max  Inputs=2
  Max1 : MinMax  Function=max  Inputs=2
  Product : Product
  Product1 : Product
  Scope : Scope
  Square{,1..3} (4 alike) : Math  Operator=square
  Square Root : Sqrt
  Square Root1 : Sqrt
  Sum : Sum  Inputs=|++
  Sum1 : Sum  Inputs=|++
  Vd\ : Outport
  Vq\ : Outport  Port=2
  wires:
  Square1/1 -> Sum/1
  Square/1 -> Sum/2
  Sum/1 -> Square Root/1
  Square Root/1 -> Max/1
  Constant/1 -> Product/2, Max/2
  Max/1 -> Divide/2
  Divide/1 -> Scope/1, Product/1
  Product/1 -> Vd\/1
  Square3/1 -> Sum1/1
  Constant1/1 -> Product1/2, Max1/2
  Square2/1 -> Sum1/2
  Divide1/1 -> Product1/1
  Vd/1 -> Square2/1, Divide/1, Square1/1
  Vq/1 -> Divide1/1, Square3/1, Square/1
  Square Root1/1 -> Max1/1
  Max1/1 -> Divide1/2
  Sum1/1 -> Square Root1/1
  Product1/1 -> Vq\/1

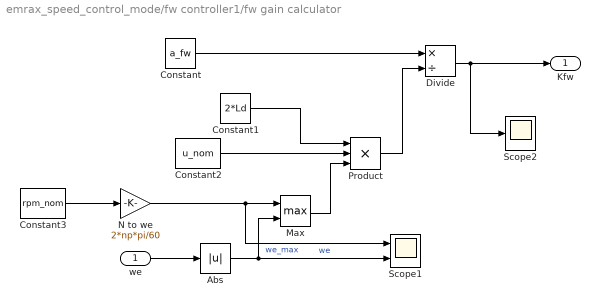
== system emrax_speed_control_mode/fw controller1/fw gain calculator ==
  we : Inport
  Abs : Abs  SaturateOnIntegerOverflow=off
  Constant : Constant  Value=a_fw
  Constant1 : Constant  Value=2*Ld
  Constant2 : Constant  Value=u_nom
  Constant3 : Constant  Value=rpm_nom
  Divide : Product  Inputs=*/
  Max : MinMax  Function=max  Inputs=2
  N to we : Gain  Gain=2*np*pi/60
  Product : Product  Inputs=3
  Scope1 : Scope  NumInputPorts=2
  Scope2 : Scope
  Kfw : Outport
  wires:
  Constant3/1 -> N to we/1
  we/1 -> Abs/1
  Abs/1 -> Max/2, Scope1/2  "we"
  Constant1/1 -> Product/1
  Constant/1 -> Divide/1
  Max/1 -> Product/3
  Constant2/1 -> Product/2
  Product/1 -> Divide/2
  Divide/1 -> Scope2/1, Kfw/1
  N to we/1 -> Scope1/1, Max/1  "we_max"

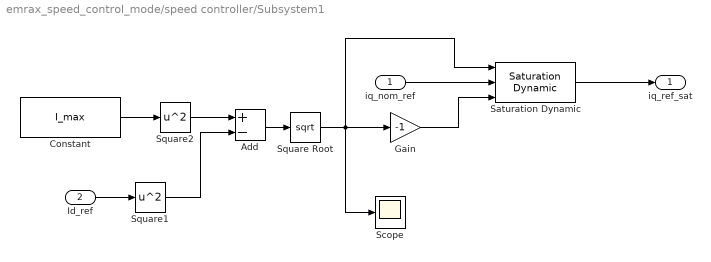
== system emrax_speed_control_mode/speed controller/Subsystem1 ==
  iq_nom_ref : Inport
  Id_ref : Inport  Port=2
  Add : Sum  Inputs=+-
  Constant : Constant  Value=I_max
  Gain : Gain  Gain=-1
  Saturation Dynamic : simulink/Discontinuities/Saturation Dynamic  OutMin=[]  OutMax=[]  OutDataTypeStr=Inherit: Same as second input  OutDataType=fixdt(1, 16)  OutScaling=2^-10  DoSatur=off
  Scope : Scope
  Square Root : Sqrt
  Square1 : Math  Operator=square
  Square2 : Math  Operator=square
  iq_ref_sat : Outport
  wires:
  Square2/1 -> Add/1
  iq_nom_ref/1 -> Saturation Dynamic/2
  Constant/1 -> Square2/1
  Square1/1 -> Add/2
  Square Root/1 -> Gain/1, Saturation Dynamic/1, Scope/1
  Add/1 -> Square Root/1
  Saturation Dynamic/1 -> iq_ref_sat/1
  Id_ref/1 -> Square1/1
  Gain/1 -> Saturation Dynamic/3
